simulink model "oscillator"  (R2014a)
settings: Solver=ode45  StartTime=0.0  StopTime=10.0  RelTol=1e-3
values from neighbouring files (symbols this model uses):
  k = 2.2e9    (= 2200000000)    [solutions406.m]
undefined symbols (not defined in the file or in its folder): b, m
settings Model: Creator=ken  LastModifiedBy=ken

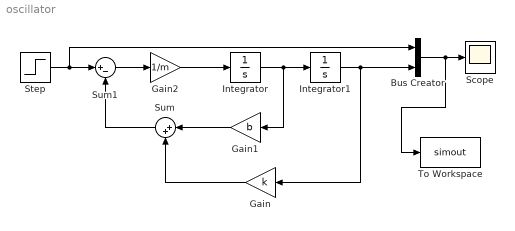
== system oscillator ==
  Bus Creator : BusCreator  Inputs=2
  Gain : Gain  Gain=k
  Gain1 : Gain  Gain=b
  Gain2 : Gain  Gain=1/m
  Integrator : Integrator
  Integrator1 : Integrator
  Scope : Scope
  Step : Step  SampleTime=0
  Sum : Sum  Inputs=|++
  Sum1 : Sum  Inputs=|+-
  To Workspace : ToWorkspace  VariableName=simout  SaveFormat=Timeseries  SampleTime=-1
  wires:
  Integrator/1 -> Gain1/1, Integrator1/1
  Integrator1/1 -> Gain/1, Bus Creator/2
  Gain/1 -> Sum/2
  Gain1/1 -> Sum/1
  Step/1 -> Bus Creator/1, Sum1/1
  Sum/1 -> Sum1/2
  Sum1/1 -> Gain2/1
  Gain2/1 -> Integrator/1
  Bus Creator/1 -> To Workspace/1, Scope/1
